simulink model "control_flow"  (R2020a)
settings: Solver=FixedStepAuto  StartTime=0.0  StopTime=5  RelTol=1e-3  EnableMultiTasking=on
settings Model: EnablePacing=on  Creator=노호진  LastModifiedBy=노호진
settings OptimizationCC: EnhancedBackFolding=on  MaxStackSize=64  OptimizeBlockOrder=speed  DifferentSizesBufferReuse=on  OptimizationCustomize=off  EfficientTunableParamExpr=on
settings DebuggingCC: ParameterTunabilityLossMsg=error
settings HardwareCC: ProdBitPerPointer=32  ProdBitPerSizeT=32  ProdBitPerPtrDiffT=32  ProdLargestAtomicInteger=Long  ProdLargestAtomicFloat=Double  ProdWordSize=32  ProdHWDeviceType=ARM Compatible->ARM Cortex
settings ModelReferenceCC: ModelReferenceNumInstancesAllowed=Zero
settings SFSimCC: SimParseCustomCode=off  MATLABDynamicMemAlloc=off
settings RTWCC: SystemTargetFile=ert.tlc  HardwareBoard=STM32F4-Discovery  TLCOptions=-aInlineSetEventsForThisBaseRateFcn=TLC_FALSE -aSuppressMultiTaskScheduler=TLC_FALSE -aRateBasedStepFcn=1  GenCodeOnly=on  TemplateMakefile=ert_default_tmf  GenerateReport=on  Toolchain=GNU Tools for ARM Embedded Processors  IncludeHyperlinkInReport=on  LaunchReport=on  GenerateTraceInfo=on  GenerateTraceReport=on  GenerateTraceReportSl=on  GenerateTraceReportSf=on  GenerateTraceReportEml=on  GenerateWebview=on  GenerateCodeMetricsReport=on
settings CodeAppCC: ForceParamTrailComments=on  IgnoreCustomStorageClasses=off  OperatorAnnotations=on  SimulinkDataObjDesc=on  SFDataObjDesc=on  InsertBlockDesc=on
settings ERTTargetCC: TargetLangStandard=C99 (ISO)  CodeReplacementLibrary=GNU C99 extensions  SuppressErrorStatus=on  SupportAbsoluteTime=off  MultiInstanceERTCode=on  CodeInterfacePackaging=Reusable function  SupportNonFinite=off  SupportComplex=off  SupportContinuousTime=on  RemoveDisableFunc=on  RootIOFormat=Part of model data structure  ERTFilePackagingFormat=Compact  ConvertIfToSwitch=off  PreserveExternInFcnDecls=off  PreserveStaticInFcnDecls=off  EnableSignedLeftShifts=off

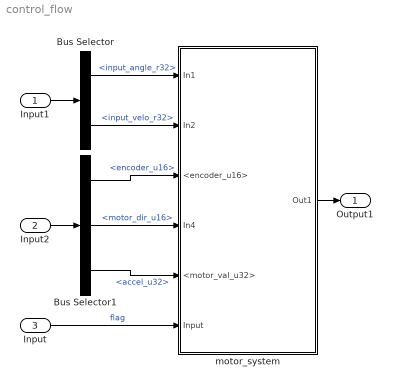
== system control_flow ==
  Input1 : Inport  OutDataTypeStr=Bus: FROM_LATTE
  Input2 : Inport  Port=2  OutDataTypeStr=Bus: MOTOR_CONTROL
  Input : Inport  Port=3  OutDataTypeStr=Bus: FROM_LATTE_FLAG
  Bus Selector : BusSelector  OutputSignals=input_angle_r32,input_velo_r32
  Bus Selector1 : BusSelector  OutputSignals=encoder_u16,motor_dir_u16,accel_u32
  motor_system : Subsystem
  Output1 : Outport  OutDataTypeStr=Bus: RETURN
  wires:
  Bus Selector1/1 -> motor_system/3(<encoder_u16>)  "<encoder_u16>"
  Bus Selector/2 -> motor_system/2(In2)  "<input_velo_r32>"
  Bus Selector/1 -> motor_system/1(In1)  "<input_angle_r32>"
  Bus Selector1/3 -> motor_system/5(<motor_val_u32>)  "<accel_u32>"
  Input2/1 -> Bus Selector1/1
  Input1/1 -> Bus Selector/1
  motor_system/1(Out1) -> Output1/1
  Bus Selector1/2 -> motor_system/4(In4)  "<motor_dir_u16>"
  Input/1 -> motor_system/6(Input)  "flag"

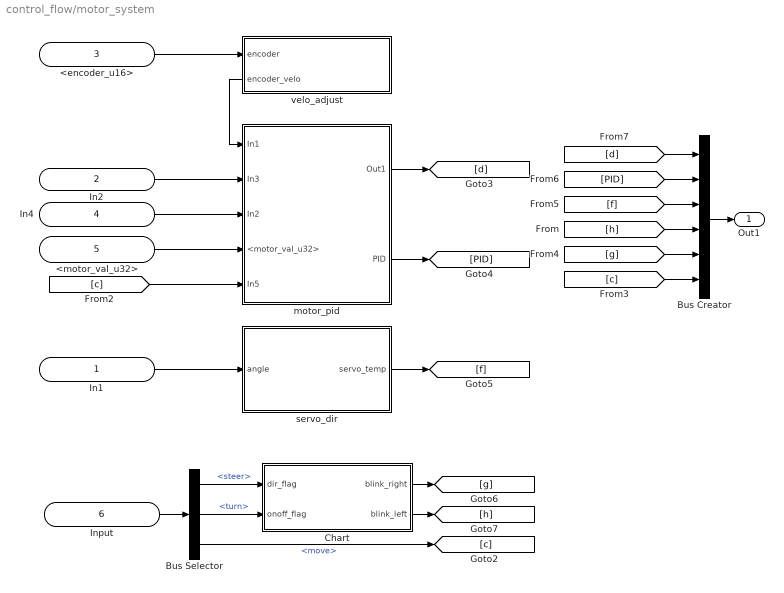
== system control_flow/motor_system ==
  In1 : Inport
  In2 : Inport  Port=2
  <encoder_u16> : Inport  Port=3
  In4 : Inport  Port=4
  <motor_val_u32> : Inport  Port=5
  Input : Inport  Port=6
  Bus Creator : BusCreator  Inputs=6  OutDataTypeStr=Bus: RETURN  NonVirtualBus=on
  Bus Selector : BusSelector  OutputSignals=steer,turn,move
  Chart : Stateflow chart  TreatAsAtomicUnit=on
  motor_pid : Subsystem
  servo_dir : Stateflow chart  TreatAsAtomicUnit=on
      settings: RTWSystemCode=Reusable function
  velo_adjust : Stateflow chart  TreatAsAtomicUnit=on
      settings: RTWSystemCode=Reusable function  PortSchema="{\"entries\":[{\"content\":{\"sides\":[{\"content\":{\"connectorIds\":[\"In1\",\"Out1\"]},\"type\":\"ConnectorPlacement.EquallySpacedRectSide\",\"uuid\":\"f5f70d90-a0f8-40b0-8904-49d6c0ee2bf6\"},{\"content\":{\"connectorIds\":[],\"side\":\"RIGHT\"},\"type\":\"ConnectorPlacement.EquallySpacedRectSide\",\"uuid\":\"467bdfc5-b9e1-4188-a769-3667078cc1c1\"},{\"content\":{\"connectorIds\":[],\"side\":\"TOP\"},\"type\":\"ConnectorPlacement.EquallySpacedRectSide\",\"uuid\":\"4f27bea3-6417-4028-8231-0b9cc6ac1b1c\"}]},\"type\":\"ConnectorPlacement.EquallySpacedConnector\",\"uuid\":\"e46cdbb7-2fa8-4e1b-80d8-26c7529314a4\"}],\"packageUris\":[\"http://schema.mathworks.com/mf0/Connector/19700101\"],\"version\":\"1.0\"}"
  Out1 : Outport
  wires:
  Bus Creator/1 -> Out1/1
  In1/1 -> servo_dir/1(angle)
  In2/1 -> motor_pid/2(In3)
  <encoder_u16>/1 -> velo_adjust/1(encoder)
  velo_adjust/1(encoder_velo) -> motor_pid/1(In1)
  <motor_val_u32>/1 -> motor_pid/4(<motor_val_u32>)
  In4/1 -> motor_pid/3(In2)
  Input/1 -> Bus Selector/1
  Bus Selector/1 -> Chart/1(dir_flag)  "<steer>"
  Bus Selector/2 -> Chart/2(onoff_flag)  "<turn>"
  Bus Selector/3 -> [c]  "<move>"
  [h] -> Bus Creator/4
  [c] -> motor_pid/5(In5)
  [c] -> Bus Creator/6
  motor_pid/1(Out1) -> [d]
  motor_pid/2(PID) -> [PID]
  servo_dir/1(servo_temp) -> [f]
  Chart/2(blink_left) -> [h]
  Chart/1(blink_right) -> [g]
  [g] -> Bus Creator/5
  [d] -> Bus Creator/1
  [PID] -> Bus Creator/2
  [f] -> Bus Creator/3

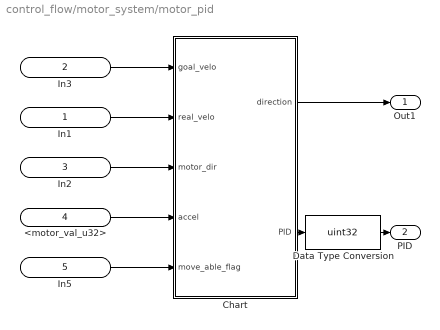
== system control_flow/motor_system/motor_pid ==
  In1 : Inport
  In3 : Inport  Port=2
  In2 : Inport  Port=3
  <motor_val_u32> : Inport  Port=4
  In5 : Inport  Port=5
  Chart : Stateflow chart  TreatAsAtomicUnit=on
  Data Type Conversion : DataTypeConversion  OutDataTypeStr=uint32
  Out1 : Outport
  PID : Outport  Port=2
  wires:
  In1/1 -> Chart/2(real_velo)
  <motor_val_u32>/1 -> Chart/4(accel)
  In2/1 -> Chart/3(motor_dir)
  Chart/1(direction) -> Out1/1
  In3/1 -> Chart/1(goal_velo)
  Chart/2(PID) -> Data Type Conversion/1
  In5/1 -> Chart/5(move_able_flag)
  Data Type Conversion/1 -> PID/1

== stateflow chart control_flow/motor_system/velo_adjust ==
  state velocity_dec
    en:
    encoder_velo = 0;
    encoder_temp = 0;
    skip_prd_cnt = 0;
    avar_velo = 0;
  state velocity_com
  (default) -> velocity_dec
  velocity_dec -> velocity_com
  (junction 64) -> velocity_com
  velocity_com -> (junction 43) : {
      | encoder_temp = encoder;
      | skip_prd_cnt++;
      | }
  (junction 43) -> (junction 24) [order 2] : [encoder_temp > MAX_uint16_T_2]
  (junction 43) -> (junction 53) [order 3]
  (junction 43) -> (junction 56) [order 1] : [encoder_temp == 0]
  (junction 24) -> (junction 53) : {encoder_temp -= MAX_uint16;}
  (junction 56) -> (junction 66) [order 2] : [encoder_velo > 0]
  (junction 56) -> (junction 68) [order 3] : [encoder_velo < 0]
  (junction 66) -> (junction 72) : {encoder_velo -= pulse_per_velo;}
  (junction 68) -> (junction 73) : {encoder_velo += pulse_per_velo;}
  (junction 56) -> (junction 64) [order 1] : {encoder_velo = (encoder_temp * pulse_per_velo) / (skip_prd_cnt * irq_prd);}
  (junction 53) -> (junction 61) : {
      | avar_velo[3] = avar_velo[2];
      | avar_velo[2] = avar_velo[1];
      | avar_velo[1] = avar_velo[0];
      | avar_velo[0] = (encoder_temp * pulse_per_velo) / (skip_prd_cnt * irq_prd);
      | encoder_velo = (avar_velo[3] + avar_velo[2] + avar_velo[1] + avar_velo[0])*0.25
      | }
  (junction 73) -> (junction 74) [order 1] : [encoder_velo > 0]
  (junction 72) -> (junction 79) [order 2]
  (junction 61) -> (junction 64) : {skip_prd_cnt = 0;}
  (junction 72) -> (junction 74) [order 1] : [encoder_velo < 0]
  (junction 73) -> (junction 79) [order 2]
  (junction 74) -> (junction 79) : {encoder_velo = 0;}
  (junction 79) -> (junction 64)
  data: encoder input; MAX_uint16_T_2 constant int32 =32767; encoder_temp local int32; MAX_uint16 constant int32 =65536; pulse_per_velo constant single =120*pi*65/744/54/2/3; irq_prd constant single =0.0005; encoder_velo output single; skip_prd_cnt local uint32; avar_velo local single size=4

== stateflow chart control_flow/motor_system/motor_pid/Chart ==
  state velo_dec
    en:
    pid_p = 0;
    pid_i = 0;
    pid_d = 0;
    PID = 0;
    direction = 0;
    err_velo = 0;
    goal_local = 0;
  state velo_com
  (default) -> velo_dec
  velo_dec -> velo_com
  (junction 108) -> velo_com
  velo_com -> (junction 118) [order 1] : [goal_velo > 300]
      | {goal_local = 300;}
  velo_com -> (junction 124) [order 3] : {goal_local = goal_velo;}
  velo_com -> (junction 122) [order 2] : [goal_velo < -300]
      | {goal_local = -300;}
  (junction 118) -> (junction 124)
  (junction 122) -> (junction 124)
  (junction 124) -> (junction 54) [order 2] : {goal_local = 0;}
  (junction 124) -> (junction 54) [order 1] : [move_able_flag == 1]
  (junction 54) -> (junction 64) : {
      | err_velo = goal_local - real_velo;
      | pid_p = err_velo;
      | pid_i += err_velo;
      | pid_d[2] = pid_d[1];
      | pid_d[1] = err_velo;
      | pid_d[0] = pid_d[2] - pid_d[1];
      | PID = goal_local + kp*pid_p + ki*pid_i + kd*pid_d[0];
      | }
  (junction 64) -> (junction 46) [order 1] : [PID > 0]
  (junction 64) -> (junction 48) [order 2] : [PID < 0]
  (junction 46) -> (junction 50) : {direction = 1;}
  (junction 64) -> (junction 44) [order 3] : {direction = motor_dir;}
  (junction 48) -> (junction 52) : {direction = 0;}
  (junction 50) -> (junction 44)
  (junction 52) -> (junction 44)
  (junction 44) -> (junction 104) : {PID = abs(PID);}
  (junction 104) -> (junction 108) [order 2]
  (junction 104) -> (junction 106) [order 1] : [PID > 1679]
  (junction 106) -> (junction 108) : {PID = 1679;}
  data: goal_velo input; real_velo input; motor_dir input; accel input; direction output uint8; err_velo local single [0..]; pid_p local single; pid_d local single size=3; pid_i local double; PID output single; kp constant double =10.0; ki constant double =1.0; kd constant double =7.5; move_able_flag input; goal_local local single

== stateflow chart control_flow/motor_system/servo_dir ==
  state angle_dec
    en:
    ang_temp = 0;
    servo_temp  = 0;
  state direction_dec
  (default) -> angle_dec
  angle_dec -> direction_dec
  direction_dec -> (junction 177) : {ang_temp = angle + 120;}
  (junction 101) -> direction_dec
  (junction 177) -> (junction 159) [order 1] : [ang_temp > ang_max]
  (junction 177) -> (junction 158) [order 2] : [ang_temp < ang_min]
  (junction 177) -> (junction 156) [order 3]
  (junction 158) -> (junction 156) : {ang_temp = ang_min;}
  (junction 159) -> (junction 156) : {ang_temp = ang_max;}
  (junction 156) -> (junction 179) : { servo_temp = (servo_prd_max - servo_prd_min)/180*ang_temp+servo_prd_min;}
  (junction 179) -> (junction 164) [order 1] : [servo_temp > servo_prd_max]
  (junction 179) -> (junction 163) [order 2] : [servo_temp < servo_prd_min]
  (junction 179) -> (junction 101) [order 3]
  (junction 163) -> (junction 101) : {servo_temp = servo_prd_min;}
  (junction 164) -> (junction 101) : {servo_temp = servo_prd_max;}
  data: angle input; ang_max constant single =150.0; ang_min constant single =90.0; ang_temp local single; servo_prd_min constant single =500/100*168; servo_prd_max constant single =2500/100*168; servo_temp output uint32

== stateflow chart control_flow/motor_system/Chart ==
  state blink_init
    en:
    blink_left = 0;
    blink_right = 0;
  state blink_com
  (default) -> blink_init
  blink_init -> blink_com
  (junction 35) -> blink_com
  blink_com -> (junction 10) [order 1] : [onoff_flag == 1]
  (junction 10) -> (junction 24) [order 1] : [dir_flag == 1]
      | {
      | blink_left = 1;
      | blink_right = 0;
      | }
  (junction 33) -> (junction 35)
  (junction 10) -> (junction 29) [order 2] : [dir_flag == 0]
      | {
      | blink_left = 0;
      | blink_right = 1;
      | }
  (junction 24) -> (junction 26)
  blink_com -> (junction 16) [order 2] : {
      | blink_left = 0;
      | blink_right = 0;
      | }
  (junction 16) -> (junction 33)
  (junction 29) -> (junction 16)
  (junction 26) -> (junction 29)
  data: dir_flag input; blink_right output uint8; blink_left output uint8; onoff_flag input
